simulink model "Dec_to_bin8_Model"  (R2024b)
settings: Solver=VariableStepAuto  StartTime=0.0  StopTime=10.0  RelTol=1e-3
libraries: NSA_DEVS_SINKS x9, NSA_DEVS_DIGITAL_CONVERTER x1, NSA_DEVS_SOURCES x1
settings Model: Creator=david  LastModifiedBy=peter
settings RTWCC: GPUComputeCapability=3.5

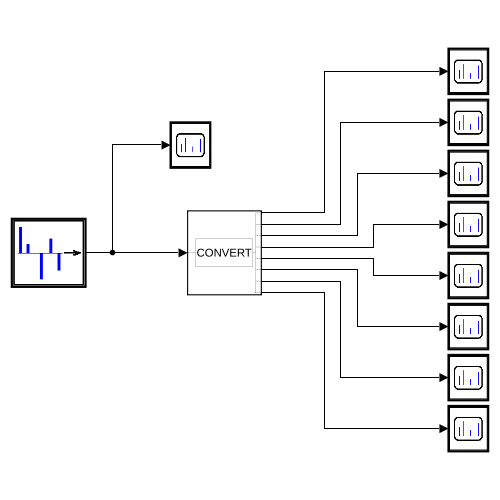
[thumbnail: Simulink's stored preview of the top-level diagram]
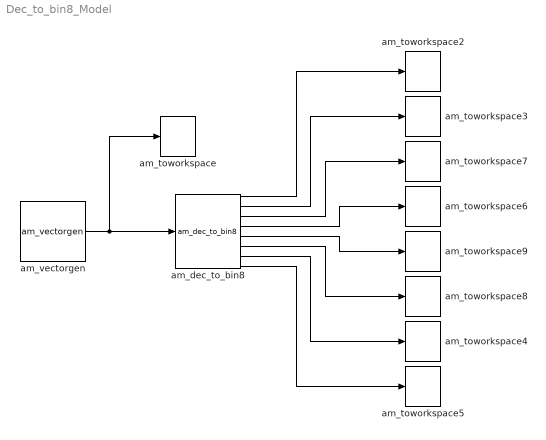
== system Dec_to_bin8_Model ==
  am_dec_to_bin8 : NSA_DEVS_DIGITAL_CONVERTER/am_dec_to_bin8  tau=[0,1]  debug=0
      settings: SourceProductName=Converter
  am_toworkspace : NSA_DEVS_SINKS/am_toworkspace  varname="\"gen1Out\""  t0=0  format="\"vector\""  tau=[0,5]  debug=0
      settings: SourceProductName=Sinks
  am_toworkspace2 : NSA_DEVS_SINKS/am_toworkspace  varname="\"dectobin8Out0\""  t0=0  format="\"vector\""  tau=[0,5]  debug=0
      settings: SourceProductName=Sinks
  am_toworkspace3 : NSA_DEVS_SINKS/am_toworkspace  varname="\"dectobin8Out1\""  t0=0  format="\"vector\""  tau=[0,5]  debug=0
      settings: SourceProductName=Sinks
  am_toworkspace4 : NSA_DEVS_SINKS/am_toworkspace  varname="\"dectobin8Out6\""  t0=0  format="\"vector\""  tau=[0,5]  debug=0
      settings: SourceProductName=Sinks
  am_toworkspace5 : NSA_DEVS_SINKS/am_toworkspace  varname="\"dectobin8Out7\""  t0=0  format="\"vector\""  tau=[0,5]  debug=0
      settings: SourceProductName=Sinks
  am_toworkspace6 : NSA_DEVS_SINKS/am_toworkspace  varname="\"dectobin8Out3\""  t0=0  format="\"vector\""  tau=[0,5]  debug=0
      settings: SourceProductName=Sinks
  am_toworkspace7 : NSA_DEVS_SINKS/am_toworkspace  varname="\"dectobin8Out2\""  t0=0  format="\"vector\""  tau=[0,5]  debug=0
      settings: SourceProductName=Sinks
  am_toworkspace8 : NSA_DEVS_SINKS/am_toworkspace  varname="\"dectobin8Out5\""  t0=0  format="\"vector\""  tau=[0,5]  debug=0
      settings: SourceProductName=Sinks
  am_toworkspace9 : NSA_DEVS_SINKS/am_toworkspace  varname="\"dectobin8Out4\""  t0=0  format="\"vector\""  tau=[0,5]  debug=0
      settings: SourceProductName=Sinks
  am_vectorgen : NSA_DEVS_SOURCES/am_vectorgen  tvec=[0:1:255]  yvec=[0:1:255]  tau=[0,1]  debug=0
      settings: SourceProductName=Sources
  wires:
  am_vectorgen/1 -> am_toworkspace/1, am_dec_to_bin8/1
  am_dec_to_bin8/1 -> am_toworkspace2/1
  am_dec_to_bin8/2 -> am_toworkspace3/1
  am_dec_to_bin8/3 -> am_toworkspace7/1
  am_dec_to_bin8/4 -> am_toworkspace6/1
  am_dec_to_bin8/5 -> am_toworkspace9/1
  am_dec_to_bin8/6 -> am_toworkspace8/1
  am_dec_to_bin8/7 -> am_toworkspace4/1
  am_dec_to_bin8/8 -> am_toworkspace5/1
